simulink model "task7_lab11"  (R2021a)
settings: Solver=VariableStepAuto  StartTime=0.0  StopTime=10.0  RelTol=1e-3
settings Model: Creator=reemb  LastModifiedBy=reemb

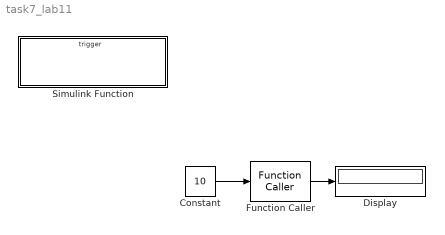
== system task7_lab11 ==
  Constant : Constant  Value=10
  Display : Display
  Function Caller : FunctionCaller  FunctionPrototype=y = multiplyByTwo(u)  InputArgumentSpecifications=<Enter example>  OutputArgumentSpecifications=<Enter example>
  Simulink Function : Subsystem  TreatAsAtomicUnit=on
  wires:
  Constant/1 -> Function Caller/1
  Function Caller/1 -> Display/1

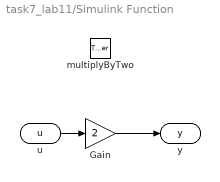
== system task7_lab11/Simulink Function ==
  multiplyByTwo : TriggerPort  TriggerType=function-call  IsSimulinkFunction=on  FunctionName=multiplyByTwo  FunctionVisibility=scoped  VariantControl=(inherit)
  Gain : Gain  Gain=2
  u : ArgIn  DisableCoverage=on  ArgumentName=u
  y : ArgOut  DisableCoverage=on  ArgumentName=y
  wires:
  u/1 -> Gain/1
  Gain/1 -> y/1
